simulink model "DC_CAR_model"  (R2022a)
settings: Solver=ode1  StartTime=0.0  StopTime=70  FixedStep=0.001  RelTol=1e-3
values from neighbouring files (symbols this model uses):
  b = 3.97e-6    (= 3.97e-06)    [DC_CAR.m]
  g = 9.81    [DC_CAR.m]    (also in sim_pendcart.m = -10)
  GR = 2.5    [DC_CAR.m]
  i_0 = 0.0    (= 0)    [DC_CAR.m]
  J = 0.0001    [DC_CAR.m]
  Kb = 0.00574    [DC_CAR.m]
  Km = Kb    (= 0.00574)    [DC_CAR.m]
  L = 0.003    [DC_CAR.m]    (also in sim_pendcart.m = 2)
  m = 1.136    [DC_CAR.m]    (also in sim_pendcart.m = 1)
  Q = 0.37    [DC_CAR.m]    (also in sim_pendcart.m = diag([1; 1; 10; 100]))
  R = 0.141    [DC_CAR.m]    (also in sim_pendcart.m = 0.1)
  Rw = 3.2e-2    (= 0.032)    [DC_CAR.m]
  tht_0 = 0.0    (= 0)    [DC_CAR.m]
  tol = 1.0e-10    (= 1e-10)    [DC_CAR.m]
  v_0 = 0.0    (= 0)    [DC_CAR.m]
  wm_0 = 0.0    (= 0)    [DC_CAR.m]
  wm_des = 275    [DC_CAR.m]
  xp_0 = 0.0    (= 0)    [DC_CAR.m]
libraries: simulink x1
settings Model: Creator=samrudh.untgodpr  LastModifiedBy=samrudh.untgodpr

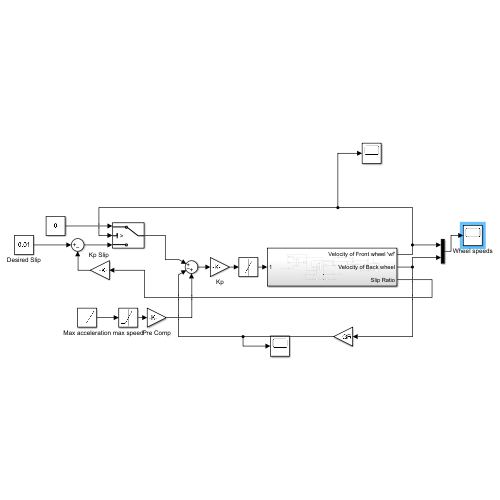
[thumbnail: Simulink's stored preview of the top-level diagram]
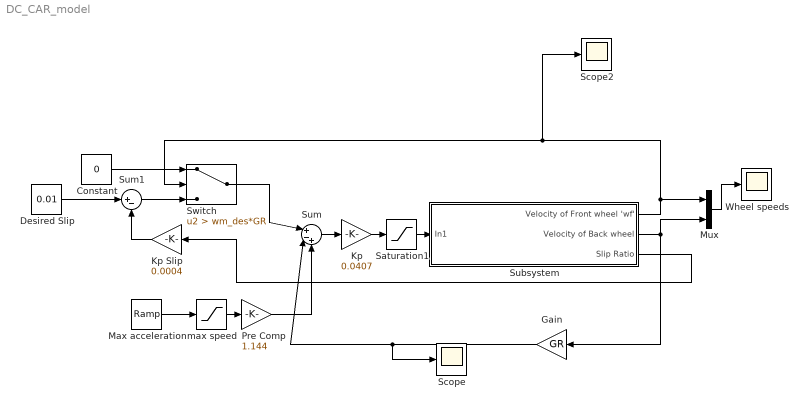
== system DC_CAR_model ==
  Constant : Constant  Value=0
  Desired Slip : Constant  Value=0.01
  Gain : Gain  Gain=GR
  Kp : Gain  Gain=0.0407
  "Kp Slip " : Gain  Gain=0.0004
  Max acceleration : simulink/Sources/Ramp  slope=50  start=0  InitialOutput=0  VectorParams1D=off
  Mux : Mux  Inputs=2
  Pre Comp : Gain  Gain=1.144
  Saturation1 : Saturate  UpperLimit=12  LowerLimit=0
  Scope : Scope
  Scope2 : Scope
  Subsystem : Subsystem
  Sum : Sum  Inputs=|+-+
  Sum1 : Sum  Inputs=|+-
  Switch : Switch  Criteria=u2 > Threshold  Threshold=wm_des*GR  SaturateOnIntegerOverflow=off  InputSameDT=off
  Wheel speeds : Scope
  max speed : Saturate  UpperLimit=wm_des  LowerLimit=0
  wires:
  Subsystem/2(Velocity of Back wheel) -> Gain/1, Mux/2
  Sum/1 -> Kp/1
  Gain/1 -> Scope/1, Sum/2
  max speed/1 -> Pre Comp/1
  Kp/1 -> Saturation1/1
  Saturation1/1 -> Subsystem/1(In1)
  Max acceleration/1 -> max speed/1
  Pre Comp/1 -> Sum/3
  Subsystem/3(Slip Ratio) -> "Kp Slip "/1
  Constant/1 -> Switch/1
  Sum1/1 -> Switch/3
  Desired Slip/1 -> Sum1/1
  "Kp Slip "/1 -> Sum1/2
  Subsystem/1(Velocity of Front wheel 'wf') -> Mux/1, Scope2/1, Switch/2
  Mux/1 -> Wheel speeds/1
  Switch/1 -> Sum/1

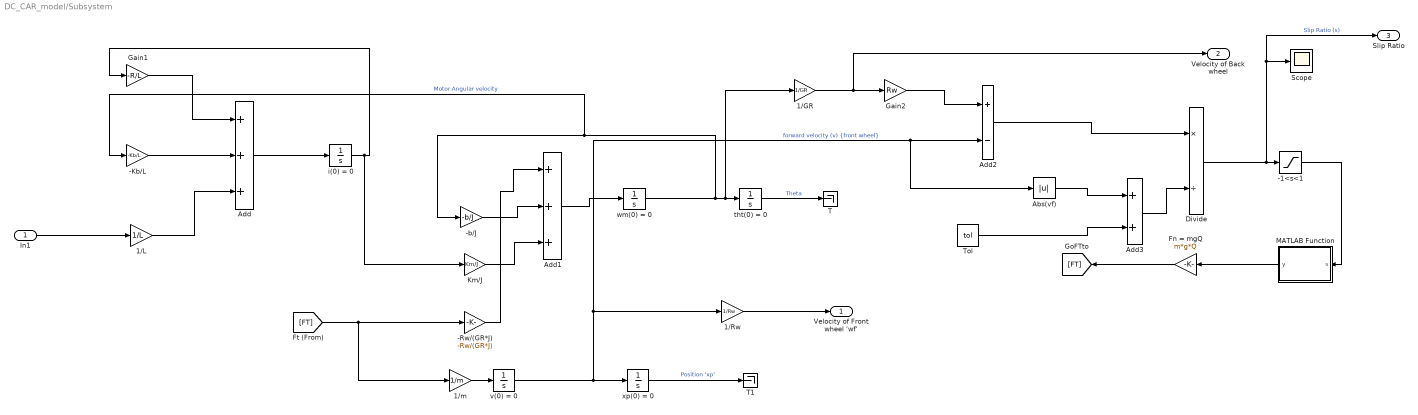
== system DC_CAR_model/Subsystem ==
  In1 : Inport
  -1<s<1 : Saturate  UpperLimit=1  LowerLimit=-1
  -Kb/L : Gain  Gain=-Kb/L
  -Rw/(GR*J) : Gain  Gain=-Rw/(GR*J)
  -b/J : Gain  Gain=-b/J
  1/GR : Gain  Gain=1/GR
  1/L : Gain  Gain=1/L
  1/Rw : Gain  Gain=1/Rw
  1/m : Gain  Gain=1/m
  Abs(vf) : Abs  SaturateOnIntegerOverflow=off
  Add : Sum  Inputs=+++
  Add1 : Sum  Inputs=+++
  Add2 : Sum  Inputs=+-
  Add3 : Sum
  Divide : Product  Inputs=*/
  Fn = mgQ : Gain  Gain=m*g*Q
  Gain1 : Gain  Gain=-R/L
  Gain2 : Gain  Gain=Rw
  Km/J : Gain  Gain=Km/J
  MATLAB Function : MATLAB Function  TreatAsAtomicUnit=on
  Scope : Scope
  T : Terminator
  T1 : Terminator
  Tol : Constant  Value=tol
  i(0) = 0 : Integrator  InitialCondition=i_0
  tht(0) = 0 : Integrator  InitialCondition=tht_0
  v(0) = 0 : Integrator  InitialCondition=v_0
  wm(0) = 0 : Integrator  InitialCondition=wm_0
  xp(0) = 0 : Integrator  InitialCondition=xp_0
  Velocity of Front wheel 'wf' : Outport
  Velocity of Back wheel : Outport  Port=2
  Slip Ratio : Outport  Port=3
  wires:
  wm(0) = 0/1 -> -Kb/L/1, -b/J/1, 1/GR/1, tht(0) = 0/1  "Motor Angular velocity"
  Abs(vf)/1 -> Add3/1
  1/m/1 -> v(0) = 0/1
  Gain1/1 -> Add/1
  v(0) = 0/1 -> xp(0) = 0/1, 1/Rw/1, Abs(vf)/1, Add2/2  "forward velocity (v) {front wheel}"
  Add1/1 -> wm(0) = 0/1
  Gain2/1 -> Add2/1
  -1<s<1/1 -> MATLAB Function/1(s)
  Fn = mgQ/1 -> [FT]
  [FT] -> 1/m/1, -Rw/(GR*J)/1
  Add/1 -> i(0) = 0/1
  Add2/1 -> Divide/1
  -b/J/1 -> Add1/2
  i(0) = 0/1 -> Km/J/1, Gain1/1
  -Rw/(GR*J)/1 -> Add1/1
  Km/J/1 -> Add1/3
  tht(0) = 0/1 -> T/1  "Theta"
  xp(0) = 0/1 -> T1/1  "Position 'xp'"
  In1/1 -> 1/L/1
  1/L/1 -> Add/3
  -Kb/L/1 -> Add/2
  1/GR/1 -> Velocity of Back wheel/1, Gain2/1
  Divide/1 -> Slip Ratio/1, Scope/1, -1<s<1/1  "Slip Ratio (s)"
  Tol/1 -> Add3/2
  Add3/1 -> Divide/2
  1/Rw/1 -> Velocity of Front wheel 'wf'/1
  MATLAB Function/1(y) -> Fn = mgQ/1

== matlab function DC_CAR_model/Subsystem/MATLAB Function ==
  data: s input; y output
function y = fcn(s)
%# codegen 
% slip is already saturated
% Only DEfined from 1 to -1

a1 = 1.63;
a2 = -0.9;
a3 = -0.1;

c1 = -27;
c2 = -15;

if s<0
    s = abs(s);
    mu = -(a1*(1-exp(c1*s))+a2*(1-exp(c2*s))+a3*s);
else
    mu =a1*(1-exp(c1*s))+a2*(1-exp(c2*s))+a3*s;
end

y = mu;
